simulink model "ex7_1"  (R2017a)
settings: Solver=ode23t  StartTime=0.0  StopTime=.3  MaxStep=1e-5  RelTol=1e-3
undefined symbols (not defined in the file): powergui, spspowerguiLib
libraries: powerlib x16, powerlib_meascontrol x4
settings Model: Creator=Omid  LastModifiedBy=Omid
settings SolverCC: ZeroCrossAlgorithm=Adaptive
settings DataIOCC: ReturnWorkspaceOutputs=on
settings OptimizationCC: LifeSpan=inf
settings DebuggingCC: IgnoredZcDiagnostic=none  UnconnectedInputMsg=none  UnconnectedOutputMsg=none  UnconnectedLineMsg=none  SFExecutionAtInitializationDiag=none
settings HardwareCC: ProdBitPerSizeT=32  ProdBitPerPtrDiffT=32  ProdWordSize=32  ProdHWDeviceType=Specified
settings SFSimCC: SimUseLocalCustomCode=on
settings RTWCC: RTWUseLocalCustomCode=on

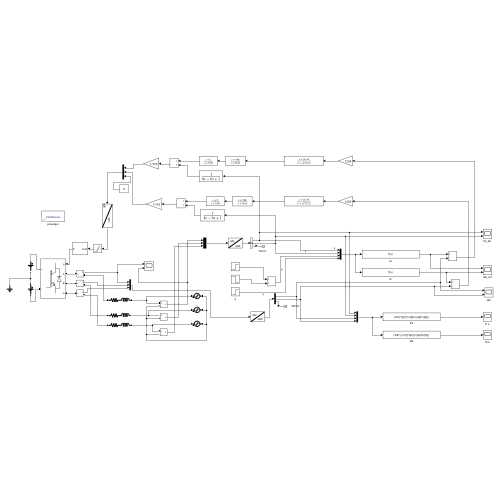
[thumbnail: Simulink's stored preview of the top-level diagram]
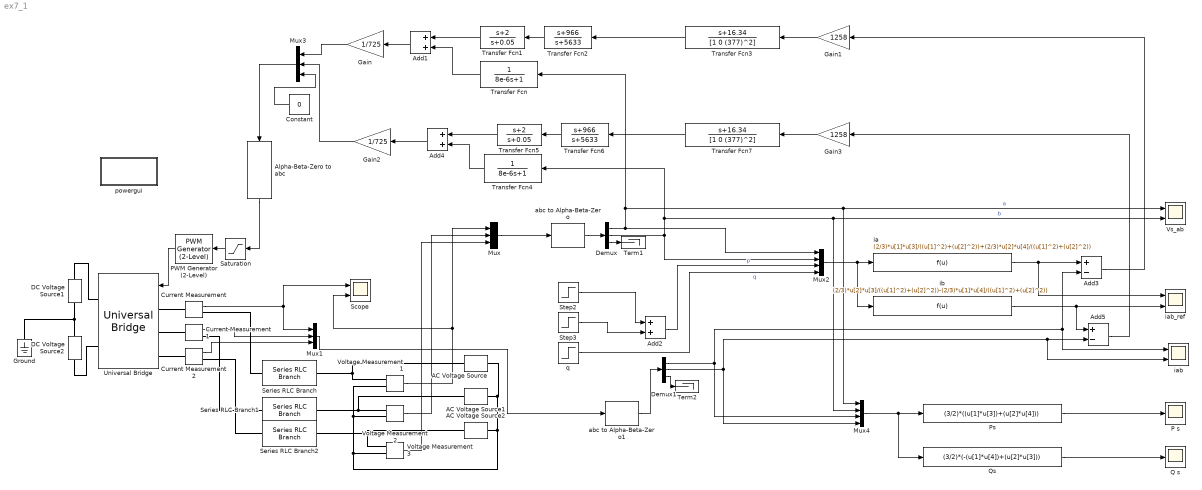
== system ex7_1 ==
  AC Voltage Source : powerlib/Electrical Sources/AC Voltage Source  Amplitude=391  Phase=0  Frequency=60  SampleTime=0  Measurements=None  BusType=swing  Pref=10e3  Qref=0  Qmin=-inf  Qmax=+inf
  AC Voltage Source1 : powerlib/Electrical Sources/AC Voltage Source  Amplitude=391  Phase=120  Frequency=60  SampleTime=0  Measurements=None  BusType=swing  Pref=10e3  Qref=0  Qmin=-inf  Qmax=+inf
  AC Voltage Source2 : powerlib/Electrical Sources/AC Voltage Source  Amplitude=391  Phase=240  Frequency=60  SampleTime=0  Measurements=None  BusType=swing  Pref=10e3  Qref=0  Qmin=-inf  Qmax=+inf
  Add1 : Sum
  Add2 : Sum
  Add3 : Sum  Inputs=+-
  Add4 : Sum
  Add5 : Sum  Inputs=+-
  Alpha-Beta-Zero to abc : powerlib_meascontrol/Transformations/Alpha-Beta-Zero to abc
  Constant : Constant  Value=0
  Current Measurement : powerlib/Measurements/Current Measurement  PhasorSimulation=off  OutputType=Complex  PSBequivalent=0
  Current Measurement1 : powerlib/Measurements/Current Measurement  PhasorSimulation=off  OutputType=Complex  PSBequivalent=0
  Current Measurement2 : powerlib/Measurements/Current Measurement  PhasorSimulation=off  OutputType=Complex  PSBequivalent=0
  DC Voltage Source1 : powerlib/Electrical Sources/DC Voltage Source  Amplitude=725  Measurements=None
  DC Voltage Source2 : powerlib/Electrical Sources/DC Voltage Source  Amplitude=725  Measurements=None
  Demux : Demux  Outputs=3
      settings: DisplayOption=none
  Demux1 : Demux  Outputs=3
  Gain : Gain  Gain=1/725
  Gain1 : Gain  Gain=1258
  Gain2 : Gain  Gain=1/725
  Gain3 : Gain  Gain=1258
  Ground : powerlib/Elements/Ground  LConnTagsString=a
  Mux : Mux  Inputs=3
  Mux1 : Mux  Inputs=3
  Mux2 : Mux
  Mux3 : Mux  Inputs=3
  Mux4 : Mux
  P s : Scope
  PWM Generator (2-Level) : powerlib_meascontrol/Pulse & Signal Generators/PWM Generator (2-Level)  ModulatorType=Three-phase bridge (6 pulses)  ModulatorMode=Unsynchronized  Fc=3420  Pc=90  nF=27  MinMax="[ -1  1 ]"  SamplingTechnique=Natural  ModulatingSignals=off  m=0.8  Freq=60  Phase=0  Ts=0  ShowCarrierOutport=off
  Ps : Fcn  Expr=(3/2)*((u[1]*u[3])+(u[2]*u[4]))
  Q s : Scope
  Qs : Fcn  Expr=(3/2)*(-(u[1]*u[4])+(u[2]*u[3]))
  Saturation : Saturate  UpperLimit=1  LowerLimit=-1
  Scope : Scope  NumInputPorts=2
  Series RLC Branch : powerlib/Elements/Series RLC Branch  LConnTagsString=__new0  RConnTagsString=__new0  BranchType=RL  Resistance=.00075  Inductance=100e-6  SetiL0=off  InitialCurrent=1600  Capacitance=1e-6  Setx0=off  InitialVoltage=0  Measurements=None
  Series RLC Branch1 : powerlib/Elements/Series RLC Branch  LConnTagsString=__new0  RConnTagsString=__new0  BranchType=RL  Resistance=.00075  Inductance=100e-6  SetiL0=off  InitialCurrent=1600  Capacitance=1e-6  Setx0=off  InitialVoltage=0  Measurements=None
  Series RLC Branch2 : powerlib/Elements/Series RLC Branch  LConnTagsString=__new0  RConnTagsString=__new0  BranchType=RL  Resistance=.00075  Inductance=100e-6  SetiL0=off  InitialCurrent=1600  Capacitance=1e-6  Setx0=off  InitialVoltage=0  Measurements=None
  Step2 : Step  Time=.1372  After=1e6  SampleTime=0
  Step3 : Step  Time=.2  After=-2e6  SampleTime=0
  Term1 : Terminator
  Term2 : Terminator
  Transfer Fcn : TransferFcn  Denominator=[8e-6 1]
  Transfer Fcn1 : TransferFcn  Numerator=[1 2]  Denominator=[1 0.05]
  Transfer Fcn2 : TransferFcn  Numerator=[1 966]  Denominator=[1 5633]
  Transfer Fcn3 : TransferFcn  Numerator=[1 16.34]  Denominator=[1 0 (377)^2]
  Transfer Fcn4 : TransferFcn  Denominator=[8e-6 1]
  Transfer Fcn5 : TransferFcn  Numerator=[1 2]  Denominator=[1 0.05]
  Transfer Fcn6 : TransferFcn  Numerator=[1 966]  Denominator=[1 5633]
  Transfer Fcn7 : TransferFcn  Numerator=[1 16.34]  Denominator=[1 0 (377)^2]
  Universal Bridge : powerlib/Power Electronics/Universal Bridge  Arms=3  SnubberResistance=1e5  SnubberCapacitance=inf  Device=IGBT / Diodes  Ron=.88e-3  Lon=0  ForwardVoltages="[  1  1 ]"  ForwardVoltage=0  GTOparameters=[ 10e-6 , 20e-6 ]  IGBTparameters=[ 1e-6 , 2e-6 ]  Measurements=None  Measurements_2=None  converterType=Rectifier
  Voltage Measurement1 : powerlib/Measurements/Voltage Measurement  PhasorSimulation=off  OutputType=Complex  PSBequivalent=0
  Voltage Measurement2 : powerlib/Measurements/Voltage Measurement  PhasorSimulation=off  OutputType=Complex  PSBequivalent=0
  Voltage Measurement3 : powerlib/Measurements/Voltage Measurement  PhasorSimulation=off  OutputType=Complex  PSBequivalent=0
  "Vs_ab " : Scope  NumInputPorts=2
  abc to Alpha-Beta-Zero : powerlib_meascontrol/Transformations/abc to Alpha-Beta-Zero
  abc to Alpha-Beta-Zero1 : powerlib_meascontrol/Transformations/abc to Alpha-Beta-Zero
  ia : Fcn  Expr=(2/3)*u[1]*u[3]/((u[1]^2)+(u[2]^2))+(2/3)*u[2]*u[4]/((u[1]^2)+(u[2]^2))
  iab : Scope  NumInputPorts=2
  iab_ref : Scope  NumInputPorts=2
  ib : Fcn  Expr=(2/3)*u[2]*u[3]/((u[1]^2)+(u[2]^2))-(2/3)*u[1]*u[4]/((u[1]^2)+(u[2]^2))
  powergui : Subsystem  Priority=1  AncestorBlock=spspowerguiLib/powergui  DialogController=POWERSYS.PowerSysDialog  InitFcn=powergui( 'InitFcn_Callback' , gcb , 0 , [ ] );  mask(PSB option menu block){SimulationMode=Continuous, SampleTime=50e-6, frequency=60, Iterations=50, frequencyindice=0, Pbase=100e6, ErrMax=1e-4, UnitsV=kV, UnitsW=MW, buscounter=0, FunctionMessages=off, echomessages=off, EnableUseOfTLC=off, CurrentSourceSwitches=off, DisableSnubberDevices=off, DisableRonSwitches=off, DisableVfSwitches=off, DisplayEquations=off, AutomaticDiscreteSolvers=off, SolverType=Tustin/Backward Euler (TBE), Interpol=off, ExternalGateDelay=off, methode=off, Ts=100, x0status=blocks, SPID=on, SwTol=0, HookPort=off, NonlinearTolerance=1e-4, nMaxIteration=100, ContinueOnMaxIteration=off, RestoreLinks=warning, ResistiveCurrentMeasurement=off, Frange=[0:2:500], Ylog=off, Xlog=on, ShowGrid=off, save=off, variable=ZData, structure=0, ZoomFFT=off, StartTime=0.0, cycles=1, DisplayStyle=1, fundamental=60, FreqAxis=off, MaxFrequency=1000, frequencyindicesteady=1, RmsSteady=1, display=off}
      mask prompts: SimulationMode "Simulation type:"; SampleTime "Sample time (s):"; frequency "Frequency (Hz):"; Iterations "Max iterations"; frequencyindice "Frequency (Hz)"; Pbase "Base power (VA)"; ErrMax "PQ tolerance (pu)"; UnitsV "Voltage units"; UnitsW "Power units"; buscounter "Load flow bus counter"; FunctionMessages "Disable Specialized Power Systems warnings"; echomessages "Display Specialized Power Systems compilation messages"; EnableUseOfTLC "Use TLC file when in Accelerator Simulation Mode and for code generation"; CurrentSourceSwitches "Disable ideal switching"; DisableSnubberDevices "Disable snubbers in switching devices"; DisableRonSwitches "Disable Ron resistances in switching devices"; DisableVfSwitches "Disable forward voltages in switching devices"; DisplayEquations "Display circuit differential equations"; AutomaticDiscreteSolvers "Automatically handle Discrete solver and Advanced tab solver settings of blocks"; SolverType "Discrete solver"; Interpol "Interpolate switching events"; ExternalGateDelay "Use time-stamped gate signals"; methode "Store switching topologies"; Ts "Buffer size (MBytes):"; x0status "Start simulation with initial electrical states from:"; SPID "Use ideal switching devices"; SwTol "Switch tolerance"; HookPort "Allow multiple powergui blocks"; NonlinearTolerance "Solver tolerance"; nMaxIteration "Maximum number of iterations"; ContinueOnMaxIteration "Continue Simulation if maximum number of iterations is reached"; RestoreLinks "Restore disabled links of Simscape Power Systems ST blocks:"; ResistiveCurrentMeasurement "Use non ideal current measurement blocks (1e-4Ohm internal resistance)"; Frange "Frequency Range"; Ylog "Log impedance"; Xlog "log Frequency"; ShowGrid "grid"; save "Save Data To Workspace"; variable "Variable Name"; structure "Structure Name (PSBFFTSCOPE)"; ZoomFFT "ZoomFFT (PSBFFTSCOPE)"; StartTime "Start Time (PSBFFTSCOPE)"; cycles "Cycles (PSBFFTSCOPE)"; DisplayStyle "Display style (PSBFFTSCOPE)"; fundamental "Fundamental (PSBFFTSCOPE)"; FreqAxis "Frequency Axis (PSBFFTSCOPE)"; MaxFrequency "Max Frequency (PSBFFTSCOPE)"; frequencyindicesteady "Frequency indice (STEADYSTATE)"; RmsSteady "RMS display (STEADYSTATE)"; display "Display Results"
      mask help: Set simulation type, simulation parameters, and preferences.
      mask init:
      | dispMessage = '';
      | dispMessage = powergui('MaskInitialization',gcb,SimulationMode,SampleTime);
      settings: PreSaveFcn=powergui( 'PreSaveFcn_Callback' , gcb , [ ] , [ ] );  OpenFcn=sps_rtmsupport('OpenFcn',gcbh)
      mask Help: helpview(psbhelp)
      mask TypeOptions SimulationMode: Continuous | Discrete | Phasor | Discrete phasor
      mask Callback SimulationMode: powergui('SimulationType',[],[],gcb);
      mask TypeOptions UnitsV: V | kV
      mask TypeOptions UnitsW: W | kW | MW
      mask Callback CurrentSourceSwitches: powergui('SimulationType',[],[],gcb);
      mask Callback AutomaticDiscreteSolvers: powergui('SimulationType',[],[],gcb);
      mask TypeOptions SolverType: Tustin/Backward Euler (TBE) | Tustin | Backward Euler
      mask Callback SolverType: powergui('SimulationType',[],[],gcb);
      mask Callback Interpol: powergui('SimulationType',[],[],gcb);
      mask Callback ExternalGateDelay: powergui('SimulationType',[],[],gcb);
      mask Callback methode: powergui('SimulationType',[],[],gcb);
      mask TypeOptions x0status: blocks | steady | zero
      mask TypeOptions RestoreLinks: yes | warning | no
      mask Callback display: sps_rtmsupport('parametereditingmodes',gcbh) % Will be executed last in parameter callbacks to ensure mask enable consistency
      mask DialogControl AutoSolverNote Prompt: The Simulation type parameter is governed by Simulink. To access the Powergui solver settings, unselect auto (Automatic solver selection) solver in the Simulink solver options.
      mask DialogControl StateAnalyzer Prompt: Measurements and States Analyzer
      mask DialogControl StateAnalyzer Callback: powerStates(bdroot(gcb))
      mask DialogControl LineParameterCalculator Prompt: Line Parameter Calculator
      mask DialogControl LineParameterCalculator Callback:
      | close_system(gcb)
      | powerLineParameters
      mask DialogControl CableParameterCalculator Prompt: Cable Parameter Calculator
      mask DialogControl CableParameterCalculator Callback:
      | close_system(gcb)
      | powerCableParameters
      mask DialogControl LineDecoupler Prompt: Line Decoupler
      mask DialogControl LineDecoupler Tooltip: Click to replace selected Distributed Parameters Line blocks with Decoupling Line blocks
      mask DialogControl LineDecoupler Callback:
      | close_system(gcb);
      | DecouplingLineReplace(gcs)
      mask DialogControl LoadFlowAnalyzer Prompt: Load Flow Analyzer
      mask DialogControl LoadFlowAnalyzer Callback:
      | close_system(gcb)
      | powerLoadFlow
      mask DialogControl LoadFlowParameters Prompt: Load Flow Parameters
      mask DialogControl ImpedanceCalculator Prompt: Impedance Calculator
      mask DialogControl ImpedanceCalculator Callback:
      | close_system(gcb);
      | powerImpedance(bdroot(gcs));
      mask DialogControl FFTAnalyzer Prompt: FFT Analyzer
      mask DialogControl FFTAnalyzer Callback:
      | close_system(gcb)
      | power_fftscope(bdroot(gcb),gcb)
      mask DialogControl LinearSystemAnalyzer Prompt: Linear System Analyzer
      mask DialogControl LinearSystemAnalyzer Callback:
      | close_system(gcb)
      | power_ltiview(bdroot(gcb))
      mask DialogControl HysteresisDesigner Prompt: Hysteresis Designer
      mask DialogControl HysteresisDesigner Callback:
      | close_system(gcb)
      | powerHysteresis('hysteresis.mat')
      mask DialogControl BlockCustomizer Prompt: Block Customizer
      mask DialogControl BlockCustomizer Callback:
      | close_system(gcb);
      | power_customize;
      mask DialogControl ReportGenerator Prompt: Report Generator
      mask DialogControl ReportGenerator Callback:
      | close_system(gcb)
      | power_report(bdroot(gcb))
      mask DialogControl obsolete Prompt: ...
      mask DialogControl MachineInitialization Prompt: Machine Initialization
      mask DialogControl MachineInitialization Callback:
      | close_system(gcb)
      | powericon('machineInitTool',bdroot(gcb),gcb)
      mask DialogControl Solver Prompt: Solver
      mask DialogControl SolverDetails Prompt: Solver details for nonlinear elements
      mask Display: color('blue'),disp(dispMessage)
  q : Step  Time=.25  After=5e5  SampleTime=0
  wires:
  Add1/1 -> Gain/1
  Voltage Measurement1/1 -> Mux/1, Scope/2
  Transfer Fcn/1 -> Add1/2
  Transfer Fcn1/1 -> Add1/1
  Add3/1 -> Gain1/1
  Transfer Fcn2/1 -> Transfer Fcn1/1
  Transfer Fcn3/1 -> Transfer Fcn2/1
  Gain1/1 -> Transfer Fcn3/1
  Voltage Measurement3/1 -> Mux/3
  Voltage Measurement2/1 -> Mux/2
  Mux/1 -> abc to Alpha-Beta-Zero/1
  abc to Alpha-Beta-Zero/1 -> Demux/1
  abc to Alpha-Beta-Zero1/1 -> Demux1/1
  Mux1/1 -> abc to Alpha-Beta-Zero1/1
  Current Measurement1/1 -> Mux1/2
  Current Measurement2/1 -> Mux1/3
  Step2/1 -> Add2/1
  Step3/1 -> Add2/2
  Demux/1 -> Transfer Fcn/1, Mux4/1, "Vs_ab "/1, Mux2/1  "a"
  Demux/2 -> Transfer Fcn4/1, Mux4/2, "Vs_ab "/2, Mux2/2  "b"
  Add2/1 -> Mux2/3  "p"
  q/1 -> Mux2/4  "q"
  Mux2/1 -> ia/1, ib/1
  ia/1 -> Add3/1, iab_ref/1
  Demux1/1 -> iab/1, Add3/2, Mux4/3
  Gain3/1 -> Transfer Fcn7/1
  Transfer Fcn7/1 -> Transfer Fcn6/1
  Transfer Fcn6/1 -> Transfer Fcn5/1
  Transfer Fcn5/1 -> Add4/1
  Transfer Fcn4/1 -> Add4/2
  Add4/1 -> Gain2/1
  Add5/1 -> Gain3/1
  ib/1 -> iab_ref/2, Add5/1
  Demux1/2 -> iab/2, Add5/2, Mux4/4
  Saturation/1 -> PWM Generator (2-Level)/1
  Gain2/1 -> Mux3/2
  Gain/1 -> Mux3/1
  PWM Generator (2-Level)/1 -> Universal Bridge/1
  Alpha-Beta-Zero to abc/1 -> Saturation/1
  Mux3/1 -> Alpha-Beta-Zero to abc/1
  Constant/1 -> Mux3/3
  Current Measurement/1 -> Mux1/1, Scope/1
  Demux1/3 -> Term2/1
  Demux/3 -> Term1/1
  Mux4/1 -> Qs/1, Ps/1
  Ps/1 -> P s/1
  Qs/1 -> Q s/1
  connections:
  DC Voltage Source1/RConn1 -- Universal Bridge/RConn1
  Current Measurement/LConn1 -- Universal Bridge/LConn1
  Series RLC Branch/LConn1 -- Current Measurement/RConn1
  Voltage Measurement1/LConn1 -- AC Voltage Source/RConn1 -- Series RLC Branch/RConn1
  Current Measurement1/LConn1 -- Universal Bridge/LConn2
  Current Measurement1/RConn1 -- Series RLC Branch1/LConn1
  Voltage Measurement2/LConn1 -- Series RLC Branch1/RConn1 -- AC Voltage Source1/RConn1
  Current Measurement2/LConn1 -- Universal Bridge/LConn3
  Series RLC Branch2/LConn1 -- Current Measurement2/RConn1
  AC Voltage Source2/RConn1 -- Series RLC Branch2/RConn1 -- Voltage Measurement3/LConn1
  DC Voltage Source2/LConn1 -- Universal Bridge/RConn2
  DC Voltage Source2/RConn1 -- Ground/LConn1 -- DC Voltage Source1/LConn1
  Voltage Measurement2/LConn2 -- AC Voltage Source/LConn1 -- AC Voltage Source1/LConn1 -- AC Voltage Source2/LConn1 -- Voltage Measurement3/LConn2 -- Voltage Measurement1/LConn2

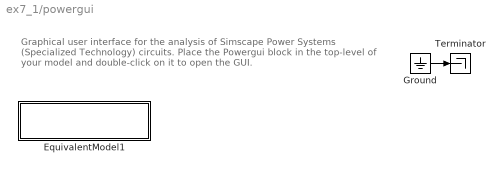
== system ex7_1/powergui ==
  note: Graphical user interface for the analysis of
      | Simscape Power Systems (Specialized Technology) circuits.
      | Place the Powergui block in the top-level of your model and double-click
      | on it to open the GUI.
  EquivalentModel1 : Subsystem  mask{SwTol=0}
      mask prompts: SwTol "SwitchTolerance"
      mask init:
      | S  = GetDataForEquivalentModel('SPID',gcbh,SwTol);
      mask Display:
      | color('blue')
      | disp('EQUIVALENT CIRCUIT\nSPID')
  Ground : Ground
  Terminator : Terminator
  wires:
  Ground/1 -> Terminator/1

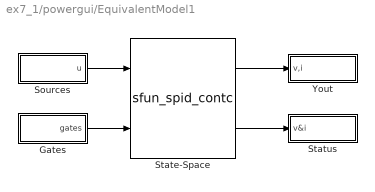
== system ex7_1/powergui/EquivalentModel1 ==
  Gates : Subsystem
  Sources : Subsystem
  State-Space : S-Function  FunctionName=sfun_spid_contc  Parameters=S.Mg, [S.nb.x S.nb.u S.nb.y S.nb.s], S.x0, S.MgColNames, S.SwitchVf, S.SwitchType, S.SwitchGateInitialValue, S.SwitchTolerance,S.SaveMatrices,S.BufferSize  SFunctionDeploymentMode=off  EnableBusSupport=off
  Status : Subsystem
  Yout : Subsystem
  wires:
  State-Space/1 -> Yout/1(v,i)
  State-Space/2 -> Status/1(v&i)
  Sources/1(u) -> State-Space/1
  Gates/1(gates) -> State-Space/2

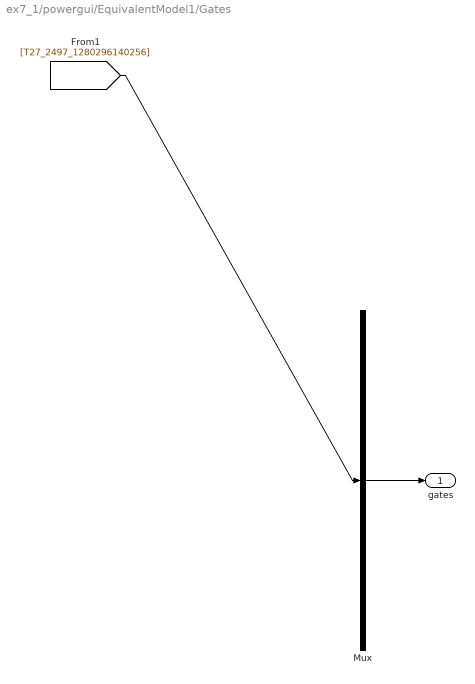
== system ex7_1/powergui/EquivalentModel1/Gates ==
  Mux : Mux  Inputs=1
  gates : Outport
  wires:
  Mux/1 -> gates/1
  [T27_2497_1280296140256] -> Mux/1

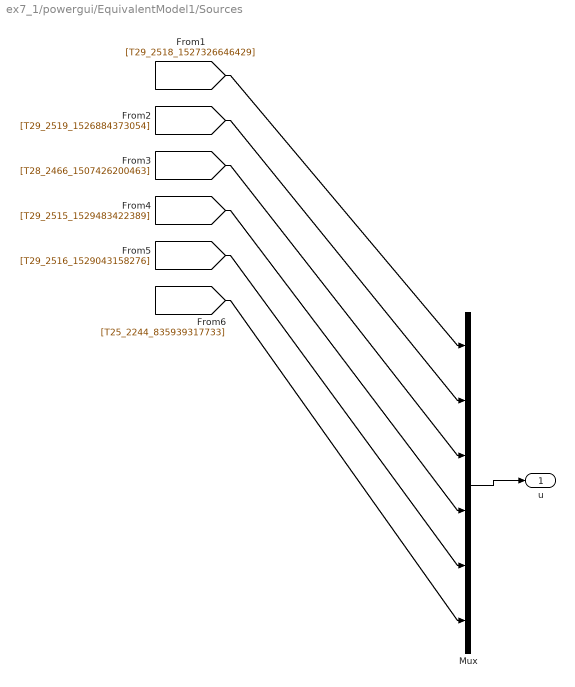
== system ex7_1/powergui/EquivalentModel1/Sources ==
  Mux : Mux  Inputs=[1 1 1 1 1 6]
  u : Outport
  wires:
  Mux/1 -> u/1
  [T29_2518_1527326646429] -> Mux/1
  [T29_2519_1526884373054] -> Mux/2
  [T28_2466_1507426200463] -> Mux/3
  [T29_2515_1529483422389] -> Mux/4
  [T29_2516_1529043158276] -> Mux/5
  [T25_2244_835939317733] -> Mux/6

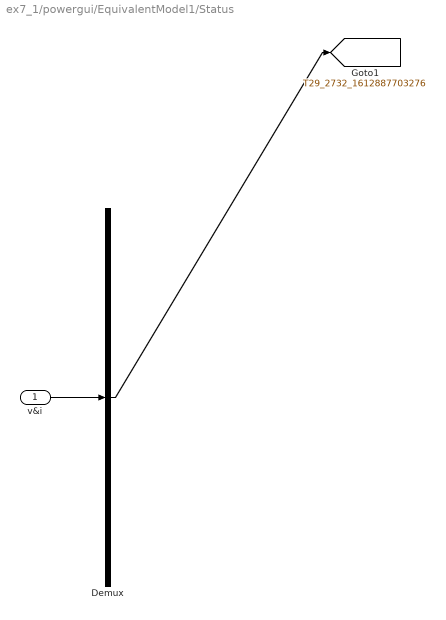
== system ex7_1/powergui/EquivalentModel1/Status ==
  v&i : Inport
  Demux : Demux  Outputs=1
  tag scope: T29_2732_1612887703276=global
  wires:
  v&i/1 -> Demux/1
  Demux/1 -> [T29_2732_1612887703276]

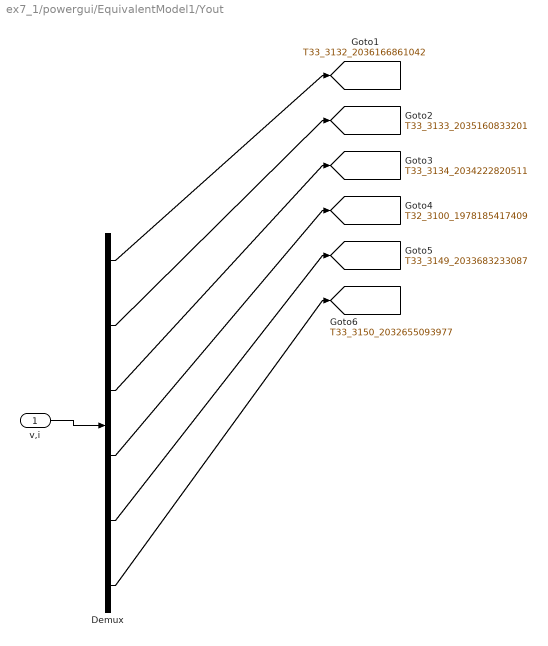
== system ex7_1/powergui/EquivalentModel1/Yout ==
  v,i : Inport
  Demux : Demux  Outputs=[1 1 1 1 1 1]
  tag scope: T32_3100_1978185417409=global, T33_3132_2036166861042=global, T33_3133_2035160833201=global, T33_3134_2034222820511=global, T33_3149_2033683233087=global, T33_3150_2032655093977=global
  wires:
  v,i/1 -> Demux/1
  Demux/1 -> [T33_3132_2036166861042]
  Demux/2 -> [T33_3133_2035160833201]
  Demux/3 -> [T33_3134_2034222820511]
  Demux/4 -> [T32_3100_1978185417409]
  Demux/5 -> [T33_3149_2033683233087]
  Demux/6 -> [T33_3150_2032655093977]
